simulink model "SFcontroleur"  (R2020a)
settings: Solver=VariableStepAuto  StartTime=0.0  StopTime=inf  RelTol=1e-3
settings Model: Creator=maxen  LastModifiedBy=maxen

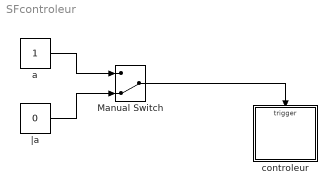
== system SFcontroleur ==
  Manual Switch : ManualSwitch  CurrentSetting=0
  a : Constant
  controleur : Stateflow chart  TreatAsAtomicUnit=on
  |a : Constant  Value=0
  wires:
  |a/1 -> Manual Switch/2
  a/1 -> Manual Switch/1
  Manual Switch/1 -> controleur/Trigger

== stateflow chart SFcontroleur/controleur ==
  settings: executeAtInitialization=1
  state On
  state Off
  On -> Off
  (default) -> Off
  Off -> On
  events: event input EITHER_EDGE_EVENT
